simulink model "MPC_Demo_wuguzhang"  (R2024a)
settings: Solver=ode1  StartTime=0.001  StopTime=16  FixedStep=0.001  RelTol=1e-3  EnableMultiTasking=on
model workspace (MAT data in the model file):
  cc = 10
libraries: simulink x3, SignalEditorBlockLib x3, Solver_SF x1, slpidlib x1
(part 3 of 5)

== matlab function MPC_Demo_wuguzhang/MATLAB Function ==
  data: Vx input; beta output; Vy input; omega_1 input; omega_2 input; omega_3 input; omega_4 input; lamda1 output; lamda2 output; lamda3 output; lamda4 output
function [beta,lamda1,lamda2,lamda3,lamda4]= fct(Vx,Vy,omega_1,omega_2,omega_3,omega_4)
beta=Vy/Vx;
Rw=0.393;
lamda1= (Rw *omega_1-Vx) / max(Vx, Rw *omega_1);
lamda2= (Rw *omega_2-Vx) / max(Vx, Rw *omega_2);
lamda3= (Rw *omega_3-Vx) / max(Vx, Rw *omega_3);
lamda4= (Rw *omega_4-Vx) / max(Vx, Rw *omega_4);

== matlab function MPC_Demo_wuguzhang/参考模型模块/质心侧偏角二阶参考模型/限幅模块 ==
  data: mu input; Vx input; beta_ref_sec output; beta_ref input; L_f input; L_r input; m input; C_f input; C_r input
function beta_ref_sec = fcn(mu,Vx,beta_ref, L_f, L_r, m, C_f, C_r)
%#codegen
% a=2*(L_f+L_r)*L_r*C_r*C_f;
% b=m*C_f*L_f*Vx^2;
% c=2*(L_f+L_r)^2*C_f*C_r-m*Vx^2*(L_f*C_f-L_r*C_r);
% beta_mid=((a-b)/c)*delta;
thre=mu*9.8*(L_r/Vx^2+m*L_f/(C_r*(L_f+L_r)));
if abs(beta_ref)>abs(thre)
    if beta_ref>=0
        beta_ref=abs(thre);
    else
        beta_ref=-abs(thre);
    end
    else
        beta_ref=beta_ref;
end

beta_ref_sec = beta_ref;

== matlab function MPC_Demo_wuguzhang/MATLAB Function2 ==
  data: Vx input; beta output; Vy input; omega_1 input; omega_2 input; omega_3 input; omega_4 input; lamda1 output; lamda2 output; lamda3 output; lamda4 output
function [beta,lamda1,lamda2,lamda3,lamda4]= fct(Vx,Vy,omega_1,omega_2,omega_3,omega_4)
beta=Vy/Vx;
Rw=0.393;
lamda1= (Rw *omega_1-Vx) / max(Vx, Rw *omega_1);
lamda2= (Rw *omega_2-Vx) / max(Vx, Rw *omega_2);
lamda3= (Rw *omega_3-Vx) / max(Vx, Rw *omega_3);
lamda4= (Rw *omega_4-Vx) / max(Vx, Rw *omega_4);
